simulink model "Utkarsh_2005574_W3_P1"  (R2020b)
settings: Solver=FixedStepDiscrete  StartTime=0.0  StopTime=180  FixedStep=0.1  RelTol=1e-3
settings Model: Creator=home  LastModifiedBy=home

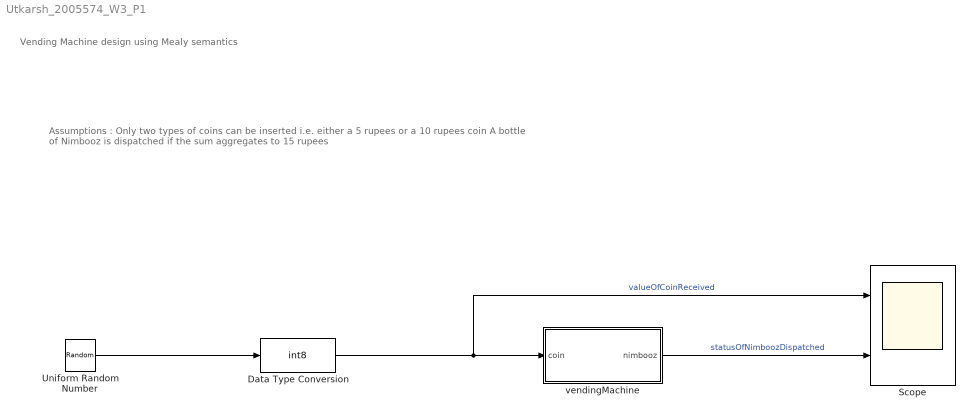
== system Utkarsh_2005574_W3_P1 ==
  note: Assumptions :
      | Only two types of coins can be inserted i.e. either a 5 rupees or a 10 rupees coin
      | A bottle of Nimbooz is dispatched if the sum aggregates to 15 rupees
  note: Vending Machine design using Mealy semantics
  Data Type Conversion : DataTypeConversion  OutDataTypeStr=int8  RndMeth=Nearest  SaturateOnIntegerOverflow=on
  Scope : Scope  NumInputPorts=2
  Uniform Random Number : UniformRandomNumber  Minimum=0  Maximum=2  Seed=337  SampleTime=10
  vendingMachine : Stateflow chart  TreatAsAtomicUnit=on
  wires:
  Uniform Random Number/1 -> Data Type Conversion/1
  Data Type Conversion/1 -> Scope/1, vendingMachine/1(coin)  "valueOfCoinReceived"
  vendingMachine/1(nimbooz) -> Scope/2  "statusOfNimboozDispatched"

== stateflow chart Utkarsh_2005574_W3_P1/vendingMachine ==
  state noCoinAvailable
  state gotTenRupeeCoin
  state gotFiveRupeeCoin
  (default) -> noCoinAvailable
  noCoinAvailable -> gotTenRupeeCoin [order 2] : [coin==2]{nimbooz=0}
  noCoinAvailable -> gotFiveRupeeCoin [order 1] : [coin==1]{nimbooz=0}
  gotTenRupeeCoin -> noCoinAvailable [order 1] : [coin==1]{nimbooz=1}
  gotFiveRupeeCoin -> noCoinAvailable [order 2] : [coin==2]{nimbooz=1}
  gotFiveRupeeCoin -> gotTenRupeeCoin [order 1] : [coin==1]{nimbooz=0}
  gotTenRupeeCoin -> gotFiveRupeeCoin [order 2] : [coin==2]{nimbooz=1}
  data: coin input; nimbooz output
